simulink library "ammclib_bam_s32k11x"  (Simulink 9.0)
settings: Solver=ode45  StartTime=0.0  StopTime=10.0  RelTol=1e-3
undefined symbols (not defined in the file): f16A1, f16A2, f16B0, f16B1, f16B2, f16C1, f16CC1, f16CC1sc, f16CC1sc_D, f16CC1sc_Q, f16CC1scD, f16CC1scQ, f16CC2, f16CC2sc, f16CC2sc_D, f16CC2sc_Q, f16CC2scD, f16CC2scQ, f16DerivGain, f16EGain, f16FiltCoef, f16HystOff, f16HystOn, f16IGain, f16IntegGain, f16IntegGainFW, f16IntegGainQ, f16Kd, f16Kq, f16Limit, f16LowerLim, f16LowerLimit_D, f16LowerLimit_Q, f16ModIndex, f16OutValOff, f16OutValOn, f16PropGain, f16PropGainFW, f16PropGainQ, f16RampDown, f16RampUp, f16UGain, f16UpperLim, f16UpperLimit, f16UpperLimit_D, f16UpperLimit_Q, f16WIGain, f32A1, f32A2, f32B0, f32B1, f32B2, f32C1, f32CC1, f32CC1sc, f32CC1sc_D, f32CC1sc_Q, f32CC1scD, f32CC1scQ, f32CC2 ... (+71)
(part 2 of 7)

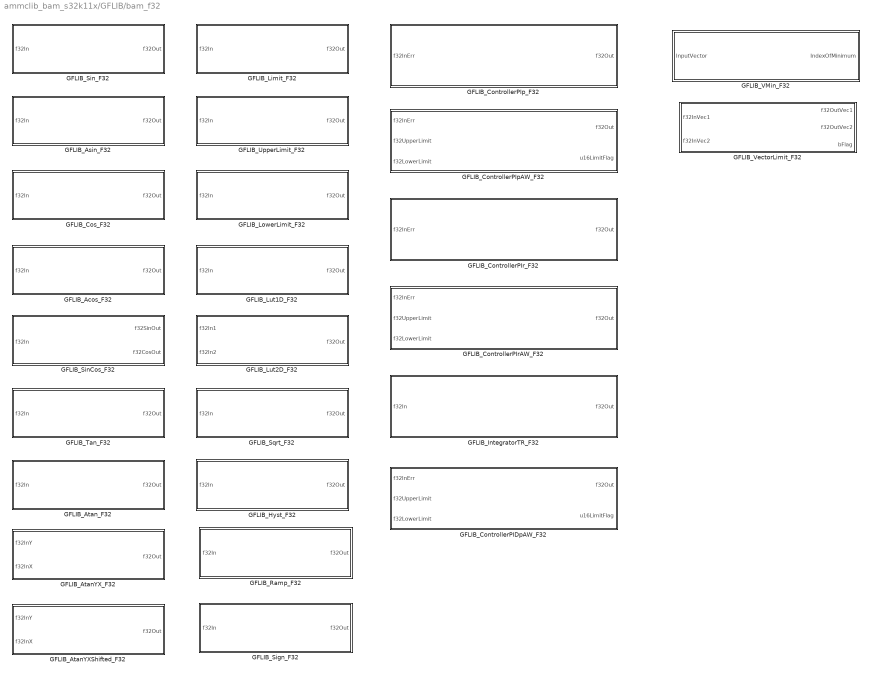
== system ammclib_bam_s32k11x/GFLIB/bam_f32 ==
  GFLIB_Acos_F32 : Subsystem  mask(GFLIB_Acos_F32){}
      mask help: Bit accurate model of GFLIB_Acos function, which computes the acos(fltIn) using the 4th order Taylor polynomial approximation.
      mask init:
      | pos = get_param(gcb, 'Position');width = pos(3) - pos(1); height = pos(4) - pos(2);tX=width/2;tY=height*0.9;
      mask Help: web(fullfile(mbd_s32k_mc_block_help('s32k11x'), 'S32K11XMCLUG.pdf'), '-browser')
      mask Display: color('black');port_label('input',1,'f32In');port_label('output',1,'f32Out');color('black');disp('GFLIB_Acos_F32');color('blue');text(tX,tY, 'BAM', 'horizontalAlignment', 'center');
  GFLIB_Asin_F32 : Subsystem  mask(GFLIB_Asin_F32){}
      mask help: Bit accurate model of GFLIB_Asin function, which computes the asin(f32In) using the 4th order Taylor polynomial approximation.
      mask init:
      | pos = get_param(gcb, 'Position');width = pos(3) - pos(1); height = pos(4) - pos(2);tX=width/2;tY=height*0.9;
      mask Help: web(fullfile(mbd_s32k_mc_block_help('s32k11x'), 'S32K11XMCLUG.pdf'), '-browser')
      mask Display: color('black');port_label('input',1,'f32In');port_label('output',1,'f32Out');color('black');disp('GFLIB_Asin_F32');color('blue');text(tX,tY, 'BAM', 'horizontalAlignment', 'center');
  GFLIB_AtanYXShifted_F32 : Subsystem  mask(GFLIB_AtanYXShifted_F32){Ky=Ky, Kx=Kx, Ny=Ny, Nx=Nx, ThetaAdj=ThetaAdj}
      mask help: Bit accurate model of GFLIB_AtanYXShifted function.
      mask init:
      | pos = get_param(gcb, 'Position');width = pos(3) - pos(1); height = pos(4) - pos(2);tX=width/2;tY=height*0.9;
      mask Help: web(fullfile(mbd_s32k_mc_block_help('s32k11x'), 'S32K11XMCLUG.pdf'), '-browser')
      mask Display: color('black');port_label('input',1,'f32InY');port_label('input',2,'f32InX');port_label('output',1,'f32Out');color('black');disp('GFLIB_AtanYXShifted_F32');color('blue');text(tX,tY, 'BAM', 'horizontalAlignment', 'center');
  GFLIB_AtanYX_F32 : Subsystem  mask(GFLIB_AtanYX_F32){}
      mask help: Bit accurate model of GFLIB_AtanYX function.
      mask init:
      | pos = get_param(gcb, 'Position');width = pos(3) - pos(1); height = pos(4) - pos(2);tX=width/2;tY=height*0.9;
      mask Help: web(fullfile(mbd_s32k_mc_block_help('s32k11x'), 'S32K11XMCLUG.pdf'), '-browser')
      mask Display: color('black');port_label('input',1,'f32InY');port_label('input',2,'f32InX');port_label('output',1,'f32Out');color('black');disp('GFLIB_AtanYX_F32');color('blue');text(tX,tY, 'BAM', 'horizontalAlignment', 'center');
  GFLIB_Atan_F32 : Subsystem  mask(GFLIB_Atan_F32){}
      mask help: Bit accurate model of GFLIB_Atan function, which computes the arctan(f32In) function.
      mask init:
      | pos = get_param(gcb, 'Position');width = pos(3) - pos(1); height = pos(4) - pos(2);tX=width/2;tY=height*0.9;
      mask Help: web(fullfile(mbd_s32k_mc_block_help('s32k11x'), 'S32K11XMCLUG.pdf'), '-browser')
      mask Display: color('black');port_label('input',1,'f32In');port_label('output',1,'f32Out');color('black');disp('GFLIB_Atan_F32');color('blue');text(tX,tY, 'BAM', 'horizontalAlignment', 'center');
  GFLIB_ControllerPIDpAW_F32 : Subsystem  mask(GFLIB_ControllerPIDpAW_F32){f32PropGain=f32PropGain, s16PropGainShift=s16PropGainShift, f32IntegGain=f32IntegGain, s16IntegGainShift=s16IntegGainShift, f32DerivGain=f32DerivGain, s16DerivGainShift=s16DerivGainShift, f32FiltCoef=f32FiltCoef}
      mask help: Bit accurate model of parallel form PID controller. All parameters as well as input and output are 32-bit integers except for s16xxxGainShift parameters which are 16-bit signed integers.
      mask init:
      | pos = get_param(gcb, 'Position');width = pos(3) - pos(1); height = pos(4) - pos(2);tX=width/2;tY=height*0.9;
      mask Display: color('black');port_label('input',1,'f32InErr');port_label('input',2,'f32UpperLimit');port_label('input',3,'f32LowerLimit');port_label('output',1,'f32Out');port_label('output',2,'u16LimitFlag');color('black');disp('GFLIB_ControllerPIDpAW_F32');color('blue');text(tX,tY, 'BAM', 'horizontalAlignment', 'center');
  GFLIB_ControllerPIpAW_F32 : Subsystem  mask(GFLIB_ControllerPIpAW_F32){f32PropGain=f32PropGain, s16PropGainShift=s16PropGainShift, f32IntegGain=f32IntegGain, s16IntegGainShift=s16IntegGainShift}
      mask help: Bit accurate model of parallel form PI controller with anti-windup. All parameters as well as input and output are 32-bit integers except for u16NShift parameter which is 16-bit unsigned integer.
      mask init:
      | pos = get_param(gcb, 'Position');width = pos(3) - pos(1); height = pos(4) - pos(2);tX=width/2;tY=height*0.9;
      mask Help: web(fullfile(mbd_s32k_mc_block_help('s32k11x'), 'S32K11XMCLUG.pdf'), '-browser')
      mask Display: color('black');port_label('input',1,'f32InErr');port_label('input',2,'f32UpperLimit');port_label('input',3,'f32LowerLimit');port_label('output',1,'f32Out');port_label('output',2,'u16LimitFlag');color('black');disp('GFLIB_ControllerPIpAW_F32');color('blue');text(tX,tY, 'BAM', 'horizontalAlignment', 'center');
  GFLIB_ControllerPIp_F32 : Subsystem  mask(GFLIB_ControllerPIp_F32){f32PropGain=f32PropGain, s16PropGainShift=s16PropGainShift, f32IntegGain=f32IntegGain, s16IntegGainShift=s16IntegGainShift}
      mask help: Bit accurate model of parallel form PI controller. All parameters as well as input and output are 32-bit integers except for u16NShift parameter which is 16-bit unsigned integer.
      mask init:
      | pos = get_param(gcb, 'Position');width = pos(3) - pos(1); height = pos(4) - pos(2);tX=width/2;tY=height*0.9;
      mask Help: web(fullfile(mbd_s32k_mc_block_help('s32k11x'), 'S32K11XMCLUG.pdf'), '-browser')
      mask Display:
      | color('black');
      | port_label('input',1,'f32InErr');
      | port_label('output',1,'f32Out');
      | color('black');
      | disp('GFLIB_ControllerPIp_F32');
      | color('blue');
      | text(tX,tY, 'BAM', 'horizontalAlignment', 'center');
  GFLIB_ControllerPIrAW_F32 : Subsystem  mask(GFLIB_ControllerPIrAW_F32){f32CC1=f32CC1, f32CC2=f32CC2, u16NShift=u16NShift}
      mask help: Bit accurate model of reccurent form PI controller with anti-windup. All parameters as well as input and output are 32-bit integers except for u16NShift parameter which is 16-bit unsigned integer.
      mask init:
      | pos = get_param(gcb, 'Position');width = pos(3) - pos(1); height = pos(4) - pos(2);tX=width/2;tY=height*0.9;
      mask Help: web(fullfile(mbd_s32k_mc_block_help('s32k11x'), 'S32K11XMCLUG.pdf'), '-browser')
      mask Display: color('black');port_label('input',1,'f32InErr');port_label('input',2,'f32UpperLimit');port_label('input',3,'f32LowerLimit');port_label('output',1,'f32Out');color('black');disp('GFLIB_ControllerPIrAW_F32');color('blue');text(tX,tY, 'BAM', 'horizontalAlignment', 'center');
  GFLIB_ControllerPIr_F32 : Subsystem  mask(GFLIB_ControllerPIr_F32){f32CC1=f32CC1, f32CC2=f32CC2, u16NShift=u16NShift}
      mask help: Bit accurate model of reccurent form PI controller. All parameters as well as input and output are 32-bit integers except for u16NShift parameter which is 16-bit unsigned integer.
      mask init:
      | pos = get_param(gcb, 'Position');width = pos(3) - pos(1); height = pos(4) - pos(2);tX=width/2;tY=height*0.9;
      mask Help: web(fullfile(mbd_s32k_mc_block_help('s32k11x'), 'S32K11XMCLUG.pdf'), '-browser')
      mask Display:
      | color('black');
      | port_label('input',1,'f32InErr');
      | port_label('output',1,'f32Out');
      | color('black');
      | disp('GFLIB_ControllerPIr_F32');
      | color('blue');
      | text(tX,tY, 'BAM', 'horizontalAlignment', 'center');
  GFLIB_Cos_F32 : Subsystem  mask(GFLIB_Cos_F32){}
      mask help: Bit accurate model of GFLIB_Cos function, which computes the cos(f32In) using the 9th order Taylor polynomial approximation.
      mask init:
      | pos = get_param(gcb, 'Position');width = pos(3) - pos(1); height = pos(4) - pos(2);tX=width/2;tY=height*0.9;
      mask Help: web(fullfile(mbd_s32k_mc_block_help('s32k11x'), 'S32K11XMCLUG.pdf'), '-browser')
      mask Display: color('black');port_label('input',1,'f32In');port_label('output',1,'f32Out');color('black');disp('GFLIB_Cos_F32');color('blue');text(tX,tY, 'BAM', 'horizontalAlignment', 'center');
  GFLIB_Hyst_F32 : Subsystem  mask(GFLIB_Hyst_F32){f32HystOn=f32HystOn, f32HystOff=f32HystOff, f32OutValOn=f32OutValOn, f32OutValOff=f32OutValOff}
      mask help: Bit accurate model of hysteresis function. All parameters as well as input and output are 32-bit integers.
      mask init:
      | pos = get_param(gcb, 'Position');width = pos(3) - pos(1); height = pos(4) - pos(2);tX=width/2;tY=height*0.9;
      mask Help: web(fullfile(mbd_s32k_mc_block_help('s32k11x'), 'S32K11XMCLUG.pdf'), '-browser')
      mask Display: color('black');port_label('input',1,'f32In');port_label('output',1,'f32Out');color('black');disp('GFLIB_Hyst_F32');color('blue');text(tX,tY, 'BAM', 'horizontalAlignment', 'center');
  GFLIB_IntegratorTR_F32 : Subsystem  mask(GFLIB_IntegratorTR_F32){f32C1=f32C1, u16NShift=u16NShift}
      mask help: Bit accurate model of discrete trapezoidal integrator. All parameters as well as input and output are full float range.
      mask init:
      | pos = get_param(gcb, 'Position');width = pos(3) - pos(1); height = pos(4) - pos(2);tX=width/2;tY=height*0.9;
      mask Help: web(fullfile(mbd_s32k_mc_block_help('s32k11x'), 'S32K11XMCLUG.pdf'), '-browser')
      mask Display:
      | color('black');
      | port_label('input',1,'f32In');
      | port_label('output',1,'f32Out');
      | color('black');
      | disp('GFLIB_IntegratorTR_F32');
      | color('blue');
      | text(tX,tY, 'BAM', 'horizontalAlignment', 'center');
  GFLIB_Limit_F32 : Subsystem  mask(GFLIB_Limit){f32UpperLimit=f32UpperLimit, f32LowerLim=f32LowerLim}
      mask help: Bit accurate model of the GFLIB_Limit function.
      mask init:
      | pos = get_param(gcb, 'Position');width = pos(3) - pos(1); height = pos(4) - pos(2);tX=width/2;tY=height*0.9;
      mask Help: web(fullfile(mbd_s32k_mc_block_help('s32k11x'), 'S32K11XMCLUG.pdf'), '-browser')
      mask Display: color('black');port_label('input',1,'f32In');port_label('output',1,'f32Out');color('black');disp('GFLIB_Limit_F32');color('blue');text(tX,tY, 'BAM', 'horizontalAlignment', 'center');
  GFLIB_LowerLimit_F32 : Subsystem  mask(GFLIB_LowerLimit_F32){f32LowerLim=f32LowerLim}
      mask help: Bit accurate model of GFLIB_LowerLimit function.
      mask init:
      | pos = get_param(gcb, 'Position');width = pos(3) - pos(1); height = pos(4) - pos(2);tX=width/2;tY=height*0.9;
      mask Help: web(fullfile(mbd_s32k_mc_block_help('s32k11x'), 'S32K11XMCLUG.pdf'), '-browser')
      mask Display: color('black');port_label('input',1,'f32In');port_label('output',1,'f32Out');color('black');disp('GFLIB_LowerLimit_F32');color('blue');text(tX,tY, 'BAM', 'horizontalAlignment', 'center');
  GFLIB_Lut1D_F32 : Subsystem  mask(GFLIB_Lut1D_F32){u32ShamOffset=u32ShamOffset, pf32Table=pf32Table, s32MidIdx=s32MidIdx}
      mask help: Bit accurate model of Lut1D function.
      mask init:
      | pos = get_param(gcb, 'Position');width = pos(3) - pos(1); height = pos(4) - pos(2);tX=width/2;tY=height*0.9;
      mask Help: web(fullfile(mbd_s32k_mc_block_help('s32k11x'), 'S32K11XMCLUG.pdf'), '-browser')
      mask Display: color('black');port_label('input',1,'f32In');port_label('output',1,'f32Out');color('black');disp('GFLIB_Lut1D_F32');color('blue');text(tX,tY, 'BAM', 'horizontalAlignment', 'center');
  GFLIB_Lut2D_F32 : Subsystem  mask(GFLIB_Lut2D_F32){u32ShamOffset1=u32ShamOffset1, u32ShamOffset2=u32ShamOffset2, pf32Table=pf32Table, s32MidIdx=s32MidIdx}
      mask help: Bit accurate model of Lut2D function.
      mask init:
      | pos = get_param(gcb, 'Position');width = pos(3) - pos(1); height = pos(4) - pos(2);tX=width/2;tY=height*0.9;
      mask Help: web(fullfile(mbd_s32k_mc_block_help('s32k11x'), 'S32K11XMCLUG.pdf'), '-browser')
      mask Display: color('black');port_label('input',1,'f32In1');port_label('input',2,'f32In2');port_label('output',1,'f32Out');color('black');disp('GFLIB_Lut2D_F32');color('blue');text(tX,tY, 'BAM', 'horizontalAlignment', 'center');
  GFLIB_Ramp_F32 : Subsystem  mask(GFLIB_Ramp){f32RampUp=f32RampUp, f32RampDown=f32RampDown}
      mask help: Bit accurate model of ramp function. All parameters as well as input and output are 32bit integers.
      mask init:
      | pos = get_param(gcb, 'Position');width = pos(3) - pos(1); height = pos(4) - pos(2);tX=width/2;tY=height*0.9;
      mask Help: web(fullfile(mbd_s32k_mc_block_help('s32k11x'), 'S32K11XMCLUG.pdf'), '-browser')
      mask Display: color('black');port_label('input',1,'f32In');port_label('output',1,'f32Out');color('black');disp('GFLIB_Ramp_F32');color('blue');text(tX,tY, 'BAM', 'horizontalAlignment', 'center');
  GFLIB_Sign_F32 : Subsystem  mask(GFLIB_Sign_F32){}
      mask help: Bit accurate model of GFLIB_Sign function.
      mask init:
      | pos = get_param(gcb, 'Position');width = pos(3) - pos(1); height = pos(4) - pos(2);tX=width/2;tY=height*0.9;
      mask Help: web(fullfile(mbd_s32k_mc_block_help('s32k11x'), 'S32K11XMCLUG.pdf'), '-browser')
      mask Display: color('black');port_label('input',1,'f32In');port_label('output',1,'f32Out');color('black');disp('GFLIB_Sign_F32');color('blue');text(tX,tY, 'BAM', 'horizontalAlignment', 'center');
  GFLIB_SinCos_F32 : Subsystem  mask(GFLIB_SinCos_F32){}
      mask help: Bit accurate model of GFLIB_SinCos function, which computes the sin(f32n) and cos(f32In) using the 9th order Taylor polynomial approximation.
      mask init:
      | pos = get_param(gcb, 'Position');width = pos(3) - pos(1); height = pos(4) - pos(2);tX=width/2;tY=height*0.9;
      mask Help: web(fullfile(mbd_s32k_mc_block_help('s32k11x'), 'S32K11XMCLUG.pdf'), '-browser')
      mask Display: color('black');port_label('input',1,'f32In');port_label('output',1,'f32SinOut');port_label('output',2,'f32CosOut');color('black');disp('GFLIB_SinCos_F32');color('blue');text(tX,tY, 'BAM', 'horizontalAlignment', 'center');
  GFLIB_Sin_F32 : Subsystem  mask(GFLIB_Sin_F32){}
      mask help: Bit accurate model of GFLIB_Sin function, which computes the sin(f32n) using the 9th order Taylor polynomial approximation.
      mask init:
      | pos = get_param(gcb, 'Position');width = pos(3) - pos(1); height = pos(4) - pos(2);tX=width/2;tY=height*0.9;
      mask Help: web(fullfile(mbd_s32k_mc_block_help('s32k11x'), 'S32K11XMCLUG.pdf'), '-browser')
      mask Display: color('black');port_label('input',1,'f32In');port_label('output',1,'f32Out');color('black');disp('GFLIB_Sin_F32');color('blue');text(tX,tY, 'BAM', 'horizontalAlignment', 'center');
  GFLIB_Sqrt_F32 : Subsystem  mask(GFLIB_Sqrt_F32){}
      mask help: Bit accurate model of GFLIB_Sqrt function, which computes the square root of input value.
      mask init:
      | pos = get_param(gcb, 'Position');width = pos(3) - pos(1); height = pos(4) - pos(2);tX=width/2;tY=height*0.9;
      mask Help: web(fullfile(mbd_s32k_mc_block_help('s32k11x'), 'S32K11XMCLUG.pdf'), '-browser')
      mask Display: color('black');port_label('input',1,'f32In');port_label('output',1,'f32Out');color('black');disp('GFLIB_Sqrt_F32');color('blue');text(tX,tY, 'BAM', 'horizontalAlignment', 'center');
  GFLIB_Tan_F32 : Subsystem  mask(GFLIB_Tan_F32){}
      mask help: Bit accurate model of GFLIB_Tan function, which computes the tan(f32In) function.
      mask init:
      | pos = get_param(gcb, 'Position');width = pos(3) - pos(1); height = pos(4) - pos(2);tX=width/2;tY=height*0.9;
      mask Help: web(fullfile(mbd_s32k_mc_block_help('s32k11x'), 'S32K11XMCLUG.pdf'), '-browser')
      mask Display: color('black');port_label('input',1,'f32In');port_label('output',1,'f32Out');color('black');disp('GFLIB_Tan_F32');color('blue');text(tX,tY, 'BAM', 'horizontalAlignment', 'center');
  GFLIB_UpperLimit_F32 : Subsystem  mask(GFLIB_UpperLimit_F32){f32UpperLim=f32UpperLim}
      mask help: Bit accurate model of GFLIB_UpperLimit function.
      mask init:
      | pos = get_param(gcb, 'Position');width = pos(3) - pos(1); height = pos(4) - pos(2);tX=width/2;tY=height*0.9;
      mask Help: web(fullfile(mbd_s32k_mc_block_help('s32k11x'), 'S32K11XMCLUG.pdf'), '-browser')
      mask Display: color('black');port_label('input',1,'f32In');port_label('output',1,'f32Out');color('black');disp('GFLIB_UpperLimit_F32');color('blue');text(tX,tY, 'BAM', 'horizontalAlignment', 'center');
  GFLIB_VMin_F32 : Subsystem  mask(GFLIB_VMin_F32){N=N}
      mask prompts: N "Vector length"
      mask help: Bit accurate model of GFLIB_VMin function, which finds the index of a vector minimum.
      mask init:
      | pos = get_param(gcb, 'Position');width = pos(3) - pos(1); height = pos(4) - pos(2);tX=width/2;tY=height*0.9;
      mask Help: web(fullfile(mbd_s32k_mc_block_help('s32k11x'), 'S32K11XMCLUG.pdf'), '-browser')
      mask Display: color('black');port_label('input',1,'InputVector');port_label('output',1,'IndexOfMinimum');color('black');disp('GFLIB_VMin_F32');color('blue');text(tX,tY, 'BAM', 'horizontalAlignment', 'center');
  GFLIB_VectorLimit_F32 : Subsystem  mask(GFLIB_VectorLimit){f32Limit=f32Limit}
      mask help: Bit accurate model of the GFLIB_VectorLimit function.
      mask init:
      | pos = get_param(gcb, 'Position');width = pos(3) - pos(1); height = pos(4) - pos(2);tX=width/2;tY=height*0.9;
      mask Help: web(fullfile(mbd_s32k_mc_block_help('s32k11x'), 'S32K11XMCLUG.pdf'), '-browser')
      mask Display: color('black');port_label('input',1,'f32InVec1');port_label('input',2,'f32InVec2');port_label('output',1,'f32OutVec1');port_label('output',2,'f32OutVec2');port_label('output',3,'bFlag');color('black');disp('GFLIB_VectorLimit_F32');color('blue');text(tX,tY, 'BAM', 'horizontalAlignment', 'center');

== system ammclib_bam_s32k11x/GMCLIB/bam_f16 ==
  GMCLIB_ClarkInv_F16 : Subsystem  mask(GMCLIB_ClarkInv_F16){}
      mask help: Bit accurate model of inverse Clarke transformation 2ph -> 3ph
      mask init:
      | pos = get_param(gcb, 'Position');width = pos(3) - pos(1); height = pos(4) - pos(2);tX=width/2;tY=height*0.9;
      mask Help: web(fullfile(mbd_s32k_mc_block_help('s32k11x'), 'S32K11XMCLUG.pdf'), '-browser')
      mask Display: color('black');port_label('input',1,'f16Alpha');port_label('input',2,'f16Beta');port_label('output',1,'f16A');port_label('output',2,'f16B');port_label('output',3,'f16C');color('black');disp('GMCLIB_ClarkInv_F16');color('blue');text(tX,tY, 'BAM', 'horizontalAlignment', 'center');
  GMCLIB_Clark_F16 : Subsystem  mask(GMCLIB_Clark_F16){}
      mask help: Bit accurate model of Clarke transformation 3ph -> 2ph.
      mask init:
      | pos = get_param(gcb, 'Position');width = pos(3) - pos(1); height = pos(4) - pos(2);tX=width/2;tY=height*0.9;
      mask Help: web(fullfile(mbd_s32k_mc_block_help('s32k11x'), 'S32K11XMCLUG.pdf'), '-browser')
      mask Display: color('black');port_label('input',1,'f16A');port_label('input',2,'f16B');port_label('input',3,'f16C');port_label('output',1,'f16Alpha');port_label('output',2,'f16Beta');color('black');disp('GMCLIB_Clark_F16');color('blue');text(tX,tY, 'BAM', 'horizontalAlignment', 'center');
  GMCLIB_DecouplingPMSM_F16 : Subsystem  mask(GMCLIB_DecouplingPMSM_F16){f16Kd=f16Kd, s16KdShift=s16KdShift, f16Kq=f16Kq, s16KqShift=s16KqShift}
      mask help: Bit accurate model of decoupling for PMSM model.
      mask init:
      | pos = get_param(gcb, 'Position');width = pos(3) - pos(1); height = pos(4) - pos(2);tX=width/2;tY=height*0.9;
      mask Help: web(fullfile(mbd_s32k_mc_block_help('s32k11x'), 'S32K11XMCLUG.pdf'), '-browser')
      mask Display: color('black');port_label('input',1,'f16Ud');port_label('input',2,'f16Uq');port_label('input',3,'f16Id');port_label('input',4,'f16Iq');port_label('input',5,'f16AngVel');port_label('output',1,'f16UdDec');port_label('output',2,'f16UqDec');color('black');disp('GMCLIB_DecouplingPMSM_F16');color('blue');text(tX,tY, 'BAM', 'horizontalAlignment', 'center');
  GMCLIB_ElimDcBusRip_F16 : Subsystem  mask(GMCLIB_ElimDcBusRip_F16){f16ModIndex=f16ModIndex}
      mask help: Bit accurate model of DC Bus voltage ripple elimination function.
      mask init:
      | pos = get_param(gcb, 'Position');width = pos(3) - pos(1); height = pos(4) - pos(2);tX=width/2;tY=height*0.9;
      mask Help: web(fullfile(mbd_s32k_mc_block_help('s32k11x'), 'S32K11XMCLUG.pdf'), '-browser')
      mask Display: color('black');port_label('input',1,'f16Alpha');port_label('input',2,'f16Beta');port_label('input',3,'f16ArgDcBusMsr');port_label('output',1,'f16AlphaOut');port_label('output',2,'f16BetaOut');color('black');disp('GMCLIB_ElimDcBusRip_F16');color('blue');text(tX,tY, 'BAM', 'horizontalAlignment', 'center');
  GMCLIB_ParkInv_F16 : Subsystem  mask(GMCLIB_ParkInv_F16){}
      mask help: Bit accurate model of Inverse Park transformation 2ph rotational -> 2ph stationary.
      mask init:
      | pos = get_param(gcb, 'Position');width = pos(3) - pos(1); height = pos(4) - pos(2);tX=width/2;tY=height*0.9;
      mask Help: web(fullfile(mbd_s32k_mc_block_help('s32k11x'), 'S32K11XMCLUG.pdf'), '-browser')
      mask Display: color('black');port_label('input',1,'f16D');port_label('input',2,'f16Q');port_label('input',3,'f16Sin');port_label('input',4,'f16Cos');port_label('output',1,'f16Alpha');port_label('output',2,'f16Beta');color('black');disp('GMCLIB_ParkInv_F16');color('blue');text(tX,tY, 'BAM', 'horizontalAlignment', 'center');
  GMCLIB_Park_F16 : Subsystem  mask(GMCLIB_Park_F16){}
      mask help: Bit accurate model of Park transformation 2ph stationary -> 2ph rotational.
      mask init:
      | pos = get_param(gcb, 'Position');width = pos(3) - pos(1); height = pos(4) - pos(2);tX=width/2;tY=height*0.9;
      mask Help: web(fullfile(mbd_s32k_mc_block_help('s32k11x'), 'S32K11XMCLUG.pdf'), '-browser')
      mask Display: color('black');port_label('input',1,'f16Alpha');port_label('input',2,'f16Beta');port_label('input',3,'f16Sin');port_label('input',4,'f16Cos');port_label('output',1,'f16D');port_label('output',2,'f16Q');color('black');disp('GMCLIB_Park_F16');color('blue');text(tX,tY, 'BAM', 'horizontalAlignment', 'center');
  GMCLIB_PwmIct_F16 : Subsystem  mask(GMCLIB_PwmIct_F16){}
      mask help: Bit accurate model of General Sinusoidal PWM.
      mask init:
      | pos = get_param(gcb, 'Position');width = pos(3) - pos(1); height = pos(4) - pos(2);tX=width/2;tY=height*0.9;
      mask Display: color('black');port_label('input',1,'f16In1');port_label('input',2,'f16In2');port_label('output',1,'f16Out1');port_label('output',2,'f16Out2');port_label('output',3,'f16Out3');port_label('output',4,'u16Sector');color('black');disp('GMCLIB_PwmIct_F16');color('blue');text(tX,tY, 'BAM', 'horizontalAlignment', 'center');
  GMCLIB_SvmStd_F16 : Subsystem  mask(GMCLIB_SvmStd_F16){}
      mask help: Bit accurate model of Standard Space Vector Modulation.
      mask init:
      | pos = get_param(gcb, 'Position');width = pos(3) - pos(1); height = pos(4) - pos(2);tX=width/2;tY=height*0.9;
      mask Help: web(fullfile(mbd_s32k_mc_block_help('s32k11x'), 'S32K11XMCLUG.pdf'), '-browser')
      mask Display: color('black');port_label('input',1,'f16In1');port_label('input',2,'f16In2');port_label('output',1,'f16Out1');port_label('output',2,'f16Out2');port_label('output',3,'f16Out3');port_label('output',4,'u16Sector');color('black');disp('GMCLIB_SvmStd_F16');color('blue');text(tX,tY, 'BAM', 'horizontalAlignment', 'center');
  GMCLIB_SvmU0n_F16 : Subsystem  mask(GMCLIB_SvmU0n_F16){}
      mask help: Bit accurate model of Standard Space Vector Modulation.
      mask init:
      | pos = get_param(gcb, 'Position');width = pos(3) - pos(1); height = pos(4) - pos(2);tX=width/2;tY=height*0.9;
      mask Display: color('black');port_label('input',1,'f16In1');port_label('input',2,'f16In2');port_label('output',1,'f16Out1');port_label('output',2,'f16Out2');port_label('output',3,'f16Out3');port_label('output',4,'u16Sector');color('black');disp('GMCLIB_SvmU0n_F16');color('blue');text(tX,tY, 'BAM', 'horizontalAlignment', 'center');

== system ammclib_bam_s32k11x/GMCLIB/bam_f32 ==
  GMCLIB_ClarkInv_F32 : Subsystem  mask(GMCLIB_ClarkInv_F32){}
      mask help: Bit accurate model of inverse Clarke transformation 2ph -> 3ph
      mask init:
      | pos = get_param(gcb, 'Position');width = pos(3) - pos(1); height = pos(4) - pos(2);tX=width/2;tY=height*0.9;
      mask Help: web(fullfile(mbd_s32k_mc_block_help('s32k11x'), 'S32K11XMCLUG.pdf'), '-browser')
      mask Display: color('black');port_label('input',1,'f32Alpha');port_label('input',2,'f32Beta');port_label('output',1,'f32A');port_label('output',2,'f32B');port_label('output',3,'f32C');color('black');disp('GMCLIB_ClarkInv_F32');color('blue');text(tX,tY, 'BAM', 'horizontalAlignment', 'center');
  GMCLIB_Clark_F32 : Subsystem  mask(GMCLIB_Clark_F32){}
      mask help: Bit accurate model of Clarke transformation 3ph -> 2ph.
      mask init:
      | pos = get_param(gcb, 'Position');width = pos(3) - pos(1); height = pos(4) - pos(2);tX=width/2;tY=height*0.9;
      mask Help: web(fullfile(mbd_s32k_mc_block_help('s32k11x'), 'S32K11XMCLUG.pdf'), '-browser')
      mask Display: color('black');port_label('input',1,'f32A');port_label('input',2,'f32B');port_label('input',3,'f32C');port_label('output',1,'f32Alpha');port_label('output',2,'f32Beta');color('black');disp('GMCLIB_Clark_F32');color('blue');text(tX,tY, 'BAM', 'horizontalAlignment', 'center');
  GMCLIB_DecouplingPMSM_F32 : Subsystem  mask(GMCLIB_DecouplingPMSM_F32){f32Kd=f32Kd, s16KdShift=s16KdShift, f32Kq=f32Kq, s16KqShift=s16KqShift}
      mask help: Bit accurate model of decoupling for PMSM model.
      mask init:
      | pos = get_param(gcb, 'Position');width = pos(3) - pos(1); height = pos(4) - pos(2);tX=width/2;tY=height*0.9;
      mask Help: web(fullfile(mbd_s32k_mc_block_help('s32k11x'), 'S32K11XMCLUG.pdf'), '-browser')
      mask Display: color('black');port_label('input',1,'f32Ud');port_label('input',2,'f32Uq');port_label('input',3,'f32Id');port_label('input',4,'f32Iq');port_label('input',5,'f32AngVel');port_label('output',1,'f32UdDec');port_label('output',2,'f32UqDec');color('black');disp('GMCLIB_DecouplingPMSM_F32');color('blue');text(tX,tY, 'BAM', 'horizontalAlignment', 'center');
  GMCLIB_ElimDcBusRip_F32 : Subsystem  mask(GMCLIB_ElimDcBusRip_F32){f32ModIndex=f32ModIndex}
      mask help: Bit accurate model of DC Bus voltage ripple elimination function.
      mask init:
      | pos = get_param(gcb, 'Position');width = pos(3) - pos(1); height = pos(4) - pos(2);tX=width/2;tY=height*0.9;
      mask Help: web(fullfile(mbd_s32k_mc_block_help('s32k11x'), 'S32K11XMCLUG.pdf'), '-browser')
      mask Display: color('black');port_label('input',1,'f32Alpha');port_label('input',2,'f32Beta');port_label('input',3,'f32ArgDcBusMsr');port_label('output',1,'f32AlphaOut');port_label('output',2,'f32BetaOut');color('black');disp('GMCLIB_ElimDcBusRip_F32');color('blue');text(tX,tY, 'BAM', 'horizontalAlignment', 'center');
  GMCLIB_ParkInv_F32 : Subsystem  mask(GMCLIB_ParkInv_F32){}
      mask help: Bit accurate model of Inverse Park transformation 2ph rotational -> 2ph stationary.
      mask init:
      | pos = get_param(gcb, 'Position');width = pos(3) - pos(1); height = pos(4) - pos(2);tX=width/2;tY=height*0.9;
      mask Help: web(fullfile(mbd_s32k_mc_block_help('s32k11x'), 'S32K11XMCLUG.pdf'), '-browser')
      mask Display: color('black');port_label('input',1,'f32D');port_label('input',2,'f32Q');port_label('input',3,'f32Sin');port_label('input',4,'f32Cos');port_label('output',1,'f32Alpha');port_label('output',2,'f32Beta');color('black');disp('GMCLIB_ParkInv_F32');color('blue');text(tX,tY, 'BAM', 'horizontalAlignment', 'center');
  GMCLIB_Park_F32 : Subsystem  mask(GMCLIB_Park_F32){}
      mask help: Bit accurate model of Park transformation 2ph stationary -> 2ph rotational.
      mask init:
      | pos = get_param(gcb, 'Position');width = pos(3) - pos(1); height = pos(4) - pos(2);tX=width/2;tY=height*0.9;
      mask Help: web(fullfile(mbd_s32k_mc_block_help('s32k11x'), 'S32K11XMCLUG.pdf'), '-browser')
      mask Display: color('black');port_label('input',1,'f32Alpha');port_label('input',2,'f32Beta');port_label('input',3,'f32Sin');port_label('input',4,'f32Cos');port_label('output',1,'f32D');port_label('output',2,'f32Q');color('black');disp('GMCLIB_Park_F32');color('blue');text(tX,tY, 'BAM', 'horizontalAlignment', 'center');
  GMCLIB_PwmIct_F32 : Subsystem  mask(GMCLIB_PwmIct_F32){}
      mask help: Bit accurate model of General Sinusoidal PWM.
      mask init:
      | pos = get_param(gcb, 'Position');width = pos(3) - pos(1); height = pos(4) - pos(2);tX=width/2;tY=height*0.9;
      mask Display: color('black');port_label('input',1,'f32In1');port_label('input',2,'f32In2');port_label('output',1,'f32Out1');port_label('output',2,'f32Out2');port_label('output',3,'f32Out3');port_label('output',4,'u32Sector');color('black');disp('GMCLIB_PwmIct_F32');color('blue');text(tX,tY, 'BAM', 'horizontalAlignment', 'center');
  GMCLIB_SvmStd_F32 : Subsystem  mask(GMCLIB_SvmStd_F32){}
      mask help: Bit accurate model of Standard Space Vector Modulation.
      mask init:
      | pos = get_param(gcb, 'Position');width = pos(3) - pos(1); height = pos(4) - pos(2);tX=width/2;tY=height*0.9;
      mask Help: web(fullfile(mbd_s32k_mc_block_help('s32k11x'), 'S32K11XMCLUG.pdf'), '-browser')
      mask Display: color('black');port_label('input',1,'f32In1');port_label('input',2,'f32In2');port_label('output',1,'f32Out1');port_label('output',2,'f32Out2');port_label('output',3,'f32Out3');port_label('output',4,'u32Sector');color('black');disp('GMCLIB_SvmStd_F32');color('blue');text(tX,tY, 'BAM', 'horizontalAlignment', 'center');
  GMCLIB_SvmU0n_F32 : Subsystem  mask(GMCLIB_SvmU0n_F32){}
      mask help: Bit accurate model of Standard Space Vector Modulation.
      mask init:
      | pos = get_param(gcb, 'Position');width = pos(3) - pos(1); height = pos(4) - pos(2);tX=width/2;tY=height*0.9;
      mask Display: color('black');port_label('input',1,'f32In1');port_label('input',2,'f32In2');port_label('output',1,'f32Out1');port_label('output',2,'f32Out2');port_label('output',3,'f32Out3');port_label('output',4,'u32Sector');color('black');disp('GMCLIB_SvmU0n_F32');color('blue');text(tX,tY, 'BAM', 'horizontalAlignment', 'center');

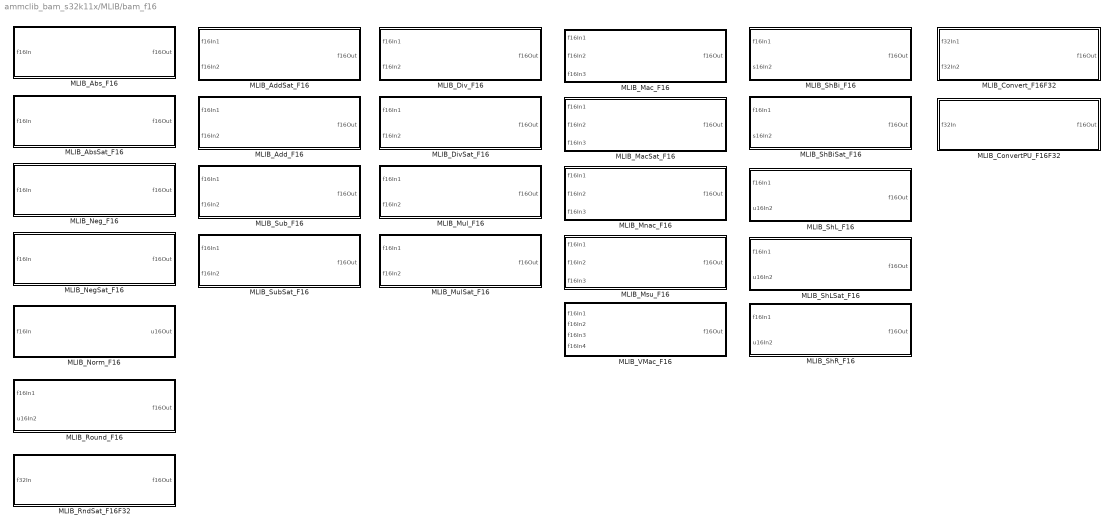
== system ammclib_bam_s32k11x/MLIB/bam_f16 ==
  MLIB_AbsSat_F16 : Subsystem  mask(MLIB_AbsSat_F16){}
      mask help: Bit accurate model for absolute value of input value. The output is saturated if necessary. All parameters as well as input and output are 16bit integers.
      mask init:
      | pos = get_param(gcb, 'Position');width = pos(3) - pos(1); height = pos(4) - pos(2);tX=width/2;tY=height*0.9;
      mask Help: web(fullfile(mbd_s32k_mc_block_help('s32k11x'), 'S32K11XMCLUG.pdf'), '-browser')
      mask Display: color('black');port_label('input',1,'f16In');port_label('output',1,'f16Out');color('black');disp('MLIB_AbsSat_F16');color('blue');text(tX,tY, 'BAM', 'horizontalAlignment', 'center');
  MLIB_Abs_F16 : Subsystem  mask(MLIB_Abs_F16){}
      mask help: Bit accurate model for absolute value of input value. All parameters as well as input and output are 16bit integers.
      mask init:
      | pos = get_param(gcb, 'Position');width = pos(3) - pos(1); height = pos(4) - pos(2);tX=width/2;tY=height*0.9;
      mask Help: web(fullfile(mbd_s32k_mc_block_help('s32k11x'), 'S32K11XMCLUG.pdf'), '-browser')
      mask Display: color('black');port_label('input',1,'f16In');port_label('output',1,'f16Out');color('black');disp('MLIB_Abs_F16');color('blue');text(tX,tY, 'BAM', 'horizontalAlignment', 'center');
  MLIB_AddSat_F16 : Subsystem  mask(MLIB_AddSat_F16){}
      mask help: Bit accurate model of saturated sum of two input values. All parameters as well as input and output are 16bit integers.
      mask init:
      | pos = get_param(gcb, 'Position');width = pos(3) - pos(1); height = pos(4) - pos(2);tX=width/2;tY=height*0.9;
      mask Help: web(fullfile(mbd_s32k_mc_block_help('s32k11x'), 'S32K11XMCLUG.pdf'), '-browser')
      mask Display: color('black');port_label('input',1,'f16In1');port_label('input',2,'f16In2');port_label('output',1,'f16Out');color('black');disp('MLIB_AddSat_F16');color('blue');text(tX,tY, 'BAM', 'horizontalAlignment', 'center');
  MLIB_Add_F16 : Subsystem  mask(MLIB_Add_F16){}
      mask help: Bit accurate model of sum of two input values. All parameters as well as input and output are 16bit integers.
      mask init:
      | pos = get_param(gcb, 'Position');width = pos(3) - pos(1); height = pos(4) - pos(2);tX=width/2;tY=height*0.9;
      mask Help: web(fullfile(mbd_s32k_mc_block_help('s32k11x'), 'S32K11XMCLUG.pdf'), '-browser')
      mask Display: color('black');port_label('input',1,'f16In1');port_label('input',2,'f16In2');port_label('output',1,'f16Out');color('black');disp('MLIB_Add_F16');color('blue');text(tX,tY, 'BAM', 'horizontalAlignment', 'center');
  MLIB_ConvertPU_F16F32 : Subsystem  mask(MLIB_ConvertPU_F16){}
      mask help: Bit accurate model for conversion value of input value. Input parameter is considered as 32-bit integer and output value is considered as 16-bit integer value.
      mask init:
      | pos = get_param(gcb, 'Position');width = pos(3) - pos(1); height = pos(4) - pos(2);tX=width/2;tY=height*0.9;
      mask Help: web(fullfile(mbd_s32k_mc_block_help('s32k11x'), 'S32K11XMCLUG.pdf'), '-browser')
      mask Display: color('black');port_label('input',1,'f32In');port_label('output',1,'f16Out');color('black');disp('MLIB_ConvertPU_F16F32');color('blue');text(tX,tY, 'BAM', 'horizontalAlignment', 'center');
  MLIB_Convert_F16F32 : Subsystem  mask(MLIB_Convert_F16F32){}
      mask help: Bit accurate model for conversion value of input value. Input parameter is considered as 32-bit integer and output value is considered as 16-bit integer value.
      mask init:
      | pos = get_param(gcb, 'Position');width = pos(3) - pos(1); height = pos(4) - pos(2);tX=width/2;tY=height*0.9;
      mask Help: web(fullfile(mbd_s32k_mc_block_help('s32k11x'), 'S32K11XMCLUG.pdf'), '-browser')
      mask Display: color('black');port_label('input',1,'f32In1');port_label('input',2,'f32In2');port_label('output',1,'f16Out');color('black');disp('MLIB_Convert_F16F32');color('blue');text(tX,tY, 'BAM', 'horizontalAlignment', 'center');
  MLIB_DivSat_F16 : Subsystem  mask(MLIB_DivSat_F16){}
      mask help: Bit accurate model of multiplication of two input values. All parameters as well as input and output are 16bit integers.
      mask init:
      | pos = get_param(gcb, 'Position');width = pos(3) - pos(1); height = pos(4) - pos(2);tX=width/2;tY=height*0.9;
      mask Help: web(fullfile(mbd_s32k_mc_block_help('s32k11x'), 'S32K11XMCLUG.pdf'), '-browser')
      mask Display: color('black');port_label('input',1,'f16In1');port_label('input',2,'f16In2');port_label('output',1,'f16Out');color('black');disp('MLIB_DivSat_F16');color('blue');text(tX,tY, 'BAM', 'horizontalAlignment', 'center');
  MLIB_Div_F16 : Subsystem  mask(MLIB_Div_F16){}
      mask help: Bit accurate model of multiplication of two input values. All parameters as well as input and output are 16bit integers.
      mask init:
      | pos = get_param(gcb, 'Position');width = pos(3) - pos(1); height = pos(4) - pos(2);tX=width/2;tY=height*0.9;
      mask Help: web(fullfile(mbd_s32k_mc_block_help('s32k11x'), 'S32K11XMCLUG.pdf'), '-browser')
      mask Display: color('black');port_label('input',1,'f16In1');port_label('input',2,'f16In2');port_label('output',1,'f16Out');color('black');disp('MLIB_Div_F16');color('blue');text(tX,tY, 'BAM', 'horizontalAlignment', 'center');
  MLIB_MacSat_F16 : Subsystem  mask(MLIB_MacSat_F16){}
      mask help: Bit accurate model of saturated multiply-accumulate of input values, staturated if necessary. All parameters as well as input and output are 16bit integers.
      mask init:
      | pos = get_param(gcb, 'Position');width = pos(3) - pos(1); height = pos(4) - pos(2);tX=width/2;tY=height*0.9;
      mask Help: web(fullfile(mbd_s32k_mc_block_help('s32k11x'), 'S32K11XMCLUG.pdf'), '-browser')
      mask Display: color('black');port_label('input',1,'f16In1');port_label('input',2,'f16In2');port_label('input',3,'f16In3');port_label('output',1,'f16Out');color('black');disp('MLIB_MacSat_F16');color('blue');text(tX,tY, 'BAM', 'horizontalAlignment', 'center');
  MLIB_Mac_F16 : Subsystem  mask(MLIB_Mac_F16){}
      mask help: Bit accurate model of multiply accumulate function. All parameters as well as input and output are 16bit integers.
      mask init:
      | pos = get_param(gcb, 'Position');width = pos(3) - pos(1); height = pos(4) - pos(2);tX=width/2;tY=height*0.9;
      mask Help: web(fullfile(mbd_s32k_mc_block_help('s32k11x'), 'S32K11XMCLUG.pdf'), '-browser')
      mask Display: color('black');port_label('input',1,'f16In1');port_label('input',2,'f16In2');port_label('input',3,'f16In3');port_label('output',1,'f16Out');color('black');disp('MLIB_Mac_F16');color('blue');text(tX,tY, 'BAM', 'horizontalAlignment', 'center');
  MLIB_Mnac_F16 : Subsystem  mask(MLIB_Mnac_F16){}
      mask help: Bit accurate model of multiply-negative-accumulate function. All parameters as well as input and output are 16bit integers.
      mask init:
      | pos = get_param(gcb, 'Position');width = pos(3) - pos(1); height = pos(4) - pos(2);tX=width/2;tY=height*0.9;
      mask Help: web(fullfile(mbd_s32k_mc_block_help('s32k11x'), 'S32K11XMCLUG.pdf'), '-browser')
      mask Display: color('black');port_label('input',1,'f16In1');port_label('input',2,'f16In2');port_label('input',3,'f16In3');port_label('output',1,'f16Out');color('black');disp('MLIB_Mnac_F16');color('blue');text(tX,tY, 'BAM', 'horizontalAlignment', 'center');
  MLIB_Msu_F16 : Subsystem  mask(MLIB_Msu_F16){}
      mask help: Bit accurate model of multiply-subtract-from function. All parameters as well as input and output are 16bit integers.
      mask init:
      | pos = get_param(gcb, 'Position');width = pos(3) - pos(1); height = pos(4) - pos(2);tX=width/2;tY=height*0.9;
      mask Help: web(fullfile(mbd_s32k_mc_block_help('s32k11x'), 'S32K11XMCLUG.pdf'), '-browser')
      mask Display: color('black');port_label('input',1,'f16In1');port_label('input',2,'f16In2');port_label('input',3,'f16In3');port_label('output',1,'f16Out');color('black');disp('MLIB_Msu_F16');color('blue');text(tX,tY, 'BAM', 'horizontalAlignment', 'center');
  MLIB_MulSat_F16 : Subsystem  mask(MLIB_MulSat_F16){}
      mask help: Bit accurate model of saturated multiplication of two input values. All parameters as well as input and output are 16bit integers.
      mask init:
      | pos = get_param(gcb, 'Position');width = pos(3) - pos(1); height = pos(4) - pos(2);tX=width/2;tY=height*0.9;
      mask Help: web(fullfile(mbd_s32k_mc_block_help('s32k11x'), 'S32K11XMCLUG.pdf'), '-browser')
      mask Display: color('black');port_label('input',1,'f16In1');port_label('input',2,'f16In2');port_label('output',1,'f16Out');color('black');disp('MLIB_MulSat_F16');color('blue');text(tX,tY, 'BAM', 'horizontalAlignment', 'center');
  MLIB_Mul_F16 : Subsystem  mask(MLIB_Mul_F16){}
      mask help: Bit accurate model of multiplication of two input values. All parameters as well as input and output are 16bit integers.
      mask init:
      | pos = get_param(gcb, 'Position');width = pos(3) - pos(1); height = pos(4) - pos(2);tX=width/2;tY=height*0.9;
      mask Help: web(fullfile(mbd_s32k_mc_block_help('s32k11x'), 'S32K11XMCLUG.pdf'), '-browser')
      mask Display: color('black');port_label('input',1,'f16In1');port_label('input',2,'f16In2');port_label('output',1,'f16Out');color('black');disp('MLIB_Mul_F16');color('blue');text(tX,tY, 'BAM', 'horizontalAlignment', 'center');
  MLIB_NegSat_F16 : Subsystem  mask(MLIB_NegSat_F16){}
      mask help: Bit accurate model for negative value of input value. The output is saturated if necessary. All parameters as well as input and output are 16bit integers.
      mask init:
      | pos = get_param(gcb, 'Position');width = pos(3) - pos(1); height = pos(4) - pos(2);tX=width/2;tY=height*0.9;
      mask Help: web(fullfile(mbd_s32k_mc_block_help('s32k11x'), 'S32K11XMCLUG.pdf'), '-browser')
      mask Display: color('black');port_label('input',1,'f16In');port_label('output',1,'f16Out');color('black');disp('MLIB_NegSat_F16');color('blue');text(tX,tY, 'BAM', 'horizontalAlignment', 'center');
  MLIB_Neg_F16 : Subsystem  mask(MLIB_Neg_F16){}
      mask help: Bit accurate model for negative value of input value. All parameters as well as input and output are 16bit integers.
      mask init:
      | pos = get_param(gcb, 'Position');width = pos(3) - pos(1); height = pos(4) - pos(2);tX=width/2;tY=height*0.9;
      mask Help: web(fullfile(mbd_s32k_mc_block_help('s32k11x'), 'S32K11XMCLUG.pdf'), '-browser')
      mask Display: color('black');port_label('input',1,'f16In');port_label('output',1,'f16Out');color('black');disp('MLIB_Neg_F16');color('blue');text(tX,tY, 'BAM', 'horizontalAlignment', 'center');
  MLIB_Norm_F16 : Subsystem  mask(MLIB_Norm_F16){}
      mask help: Bit accurate model of the normalization function. The function counts the number of left shift needed for normalization of the input fractional value.
      mask init:
      | pos = get_param(gcb, 'Position');width = pos(3) - pos(1); height = pos(4) - pos(2);tX=width/2;tY=height*0.9;
      mask Help: web(fullfile(mbd_s32k_mc_block_help('s32k11x'), 'S32K11XMCLUG.pdf'), '-browser')
      mask Display: color('black');port_label('input',1,'f16In');port_label('output',1,'u16Out');color('black');disp('MLIB_Norm_F16');color('blue');text(tX,tY, 'BAM', 'horizontalAlignment', 'center');
  MLIB_RndSat_F16F32 : Subsystem  mask(MLIB_RndSat_F16F32){}
      mask help: Bit accurate model for conversion of input value. Input parameter is considered as 32-bit integer and output value is considered as 16-bit integer value.
      mask init:
      | pos = get_param(gcb, 'Position');width = pos(3) - pos(1); height = pos(4) - pos(2);tX=width/2;tY=height*0.9;
      mask Help: web(fullfile(mbd_s32k_mc_block_help('s32k11x'), 'S32K11XMCLUG.pdf'), '-browser')
      mask Display: color('black');port_label('input',1,'f32In');port_label('output',1,'f16Out');color('black');disp('MLIB_RndSat_F16F32');color('blue');text(tX,tY, 'BAM', 'horizontalAlignment', 'center');
  MLIB_Round_F16 : Subsystem  mask(MLIB_Round_F16){}
      mask help: Bit accurate model of the fuction rounds the first input value for number of digits defined by second parameter and saturate automaticaly. All parameters as well as input and output are 16bit integers.
      mask init:
      | pos = get_param(gcb, 'Position');width = pos(3) - pos(1); height = pos(4) - pos(2);tX=width/2;tY=height*0.9;
      mask Help: web(fullfile(mbd_s32k_mc_block_help('s32k11x'), 'S32K11XMCLUG.pdf'), '-browser')
      mask Display: color('black');port_label('input',1,'f16In1');port_label('input',2,'u16In2');port_label('output',1,'f16Out');color('black');disp('MLIB_Round_F16');color('blue');text(tX,tY, 'BAM', 'horizontalAlignment', 'center');
  MLIB_ShBiSat_F16 : Subsystem  mask(MLIB_ShBiSat_F16){}
      mask help: Bit accurate model of the fuction shifts the first parameter to left or right by number defined by second parameter and saturate if necessary. If the sign of second parameter is negative, shift to right. All parameters as well as input and output are 16bit integers.
      mask init:
      | pos = get_param(gcb, 'Position');width = pos(3) - pos(1); height = pos(4) - pos(2);tX=width/2;tY=height*0.9;
      mask Help: web(fullfile(mbd_s32k_mc_block_help('s32k11x'), 'S32K11XMCLUG.pdf'), '-browser')
      mask Display: color('black');port_label('input',1,'f16In1');port_label('input',2,'s16In2');port_label('output',1,'f16Out');color('black');disp('MLIB_ShBiSat_F16');color('blue');text(tX,tY, 'BAM', 'horizontalAlignment', 'center');
  MLIB_ShBi_F16 : Subsystem  mask(MLIB_ShBi_F16){}
      mask help: Bit accurate model of the fuction shifts the first parameter to left or right by number defined by second parameter. If the sign of second parameter is negative, shift to right. All parameters as well as input and output are 16bit integers.
      mask init:
      | pos = get_param(gcb, 'Position');width = pos(3) - pos(1); height = pos(4) - pos(2);tX=width/2;tY=height*0.9;
      mask Help: web(fullfile(mbd_s32k_mc_block_help('s32k11x'), 'S32K11XMCLUG.pdf'), '-browser')
      mask Display: color('black');port_label('input',1,'f16In1');port_label('input',2,'s16In2');port_label('output',1,'f16Out');color('black');disp('MLIB_ShBi_F16');color('blue');text(tX,tY, 'BAM', 'horizontalAlignment', 'center');
  MLIB_ShLSat_F16 : Subsystem  mask(MLIB_ShLSat_F16){}
      mask help: Bit accurate model of the fuction shifts the first parameter to left by number defined by second parameter and saturate if necessary. All parameters as well as input and output are 16bit integers.
      mask init:
      | pos = get_param(gcb, 'Position');width = pos(3) - pos(1); height = pos(4) - pos(2);tX=width/2;tY=height*0.9;
      mask Help: web(fullfile(mbd_s32k_mc_block_help('s32k11x'), 'S32K11XMCLUG.pdf'), '-browser')
      mask Display: color('black');port_label('input',1,'f16In1');port_label('input',2,'u16In2');port_label('output',1,'f16Out');color('black');disp('MLIB_ShLSat_F16');color('blue');text(tX,tY, 'BAM', 'horizontalAlignment', 'center');
  MLIB_ShL_F16 : Subsystem  mask(MLIB_ShL_F16){}
      mask help: Bit accurate model of the fuction shifts the first parameter to left by number defined by second parameter. All parameters as well as input and output are 16bit integers.
      mask init:
      | pos = get_param(gcb, 'Position');width = pos(3) - pos(1); height = pos(4) - pos(2);tX=width/2;tY=height*0.9;
      mask Help: web(fullfile(mbd_s32k_mc_block_help('s32k11x'), 'S32K11XMCLUG.pdf'), '-browser')
      mask Display: color('black');port_label('input',1,'f16In1');port_label('input',2,'u16In2');port_label('output',1,'f16Out');color('black');disp('MLIB_ShL_F16');color('blue');text(tX,tY, 'BAM', 'horizontalAlignment', 'center');
  MLIB_ShR_F16 : Subsystem  mask(MLIB_ShR_F16){}
      mask help: Bit accurate model of the fuction shifts the first parameter to right by number defined by second parameter. All parameters as well as input and output are 16bit integers.
      mask init:
      | pos = get_param(gcb, 'Position');width = pos(3) - pos(1); height = pos(4) - pos(2);tX=width/2;tY=height*0.9;
      mask Help: web(fullfile(mbd_s32k_mc_block_help('s32k11x'), 'S32K11XMCLUG.pdf'), '-browser')
      mask Display: color('black');port_label('input',1,'f16In1');port_label('input',2,'u16In2');port_label('output',1,'f16Out');color('black');disp('MLIB_ShR_F16');color('blue');text(tX,tY, 'BAM', 'horizontalAlignment', 'center');
  MLIB_SubSat_F16 : Subsystem  mask(MLIB_SubSat_F16){}
      mask help: Bit accurate model of saturated subtraction of two input values. All parameters as well as input and output are 16bit integers.
      mask init:
      | pos = get_param(gcb, 'Position');width = pos(3) - pos(1); height = pos(4) - pos(2);tX=width/2;tY=height*0.9;
      mask Help: web(fullfile(mbd_s32k_mc_block_help('s32k11x'), 'S32K11XMCLUG.pdf'), '-browser')
      mask Display: color('black');port_label('input',1,'f16In1');port_label('input',2,'f16In2');port_label('output',1,'f16Out');color('black');disp('MLIB_SubSat_F16');color('blue');text(tX,tY, 'BAM', 'horizontalAlignment', 'center');
  MLIB_Sub_F16 : Subsystem  mask(MLIB_Sub_F16){}
      mask help: Bit accurate model of subtract of two input values. All parameters as well as input and output are 16bit integers.
      mask init:
      | pos = get_param(gcb, 'Position');width = pos(3) - pos(1); height = pos(4) - pos(2);tX=width/2;tY=height*0.9;
      mask Help: web(fullfile(mbd_s32k_mc_block_help('s32k11x'), 'S32K11XMCLUG.pdf'), '-browser')
      mask Display: color('black');port_label('input',1,'f16In1');port_label('input',2,'f16In2');port_label('output',1,'f16Out');color('black');disp('MLIB_Sub_F16');color('blue');text(tX,tY, 'BAM', 'horizontalAlignment', 'center');
  MLIB_VMac_F16 : Subsystem  mask(MLIB_VMac_F16){}
      mask help: Bit accurate model of vector multiply accumulate function. All parameters as well as input and output are 16-bit integers.
      mask init:
      | pos = get_param(gcb, 'Position');width = pos(3) - pos(1); height = pos(4) - pos(2);tX=width/2;tY=height*0.9;
      mask Help: web(fullfile(mbd_s32k_mc_block_help('s32k11x'), 'S32K11XMCLUG.pdf'), '-browser')
      mask Display: color('black');port_label('input',1,'f16In1');port_label('input',2,'f16In2');port_label('input',3,'f16In3');port_label('input',4,'f16In4');port_label('output',1,'f16Out');color('black');disp('MLIB_VMac_F16');color('blue');text(tX,tY, 'BAM', 'horizontalAlignment', 'center');
